simulink model "Vehicle_Model_Controller_Feb25"  (R2020b)
settings: Solver=VariableStepAuto  StartTime=0.0  StopTime=60  FixedStep=0.015  MaxStep=0.015  RelTol=1e-3
model workspace (MAT data in the model file):
  Kp = 10
  understeer_gradient = 0.05
values from neighbouring files (symbols this model uses):
  I = 0    [startup.m]
  P = 10    [startup.m]
  T = 0    [startup.m]
undefined symbols (not defined in the file or in its folder): DiscIntNeverNeededParam
libraries: fl_lib x32, nesl_utility x24, sdl_lib x8, vehdynlibsteering x1, autolibshared x1, autolibdatasheetbattery x1, pid_lib x1
(part 1 of 3)
settings Model: TunableVars=F_sv,F_x_ij,F_x_ij_max,F_y_fl,F_y_fr,F_y_ij,F_y_rl,F_y_rr,J_z,K_1,K_2,LB,PID,R,T_x_ij,UP,delta,driver_input,err,l,l_f,l_r,linsol,s,s_f,s_r,x,x_1,x_2,x_3,x_4,y,y_1,y_2,y_3,y_4  TunableVarsStorageClass=Auto,Auto,Auto,Auto,Auto,Auto,Auto,Auto,Auto,Auto,Auto,Auto,Auto,Auto,Auto,Auto,Auto,Auto,Auto,Auto,Auto,Auto,Auto,Auto,Auto,Auto,Auto,Auto,Auto,Auto,Auto,Auto,Auto,Auto,Auto,Auto  TunableVarsTypeQualifier=,,,,,,,,,,,,,,,,,,,,,,,,,,,,,,,,,,,  ParameterArgumentNames=understeer_gradient  OrderedModelArguments=off  Creator=True  LastModifiedBy=Inver
settings SolverCC: MaxConsecutiveMinStep=10  AutoInsertRateTranBlk=on  MinimalZcImpactIntegration=on
settings DataIOCC: ExternalInput=Sheet1.getElement('driver_input'),Sheet1.getElement('P_A'),Sheet1.getElement('B_A'),Sheet1.getElement('steering_angle'),Sheet1.getElement('wind x'),Sheet1.getElement('wind y'),Sheet1.getElement('wind z'),Sheet1.getElement('batt_temp')  LoadExternalInput=on
settings OptimizationCC: DefaultParameterBehavior=Inlined  UseFloatMulNetSlope=on  InlineInvariantSignals=on  BufferReuse=off  EnhancedBackFolding=on  PassReuseOutputArgsThreshold=0  EfficientFloat2IntCast=on  EfficientMapNaN2IntZero=off  OptimizeBlockOrder=speed  DifferentSizesBufferReuse=on
settings DebuggingCC: RTPrefix=warning  ReadBeforeWriteMsg=DisableAll  WriteAfterWriteMsg=DisableAll  WriteAfterReadMsg=DisableAll  SolverPrmCheckMsg=error  MultiTaskDSMMsg=none  ParameterTunabilityLossMsg=error  ArithmeticOperatorsInVariantConditions=warning
settings HardwareCC: TargetBitPerPointer=64  TargetBitPerSizeT=64  TargetBitPerPtrDiffT=64  TargetLongLongMode=on  TargetIntDivRoundTo=Zero  TargetEndianess=LittleEndian  TargetWordSize=64  TargetHWDeviceType=MATLAB Host  ProdEqTarget=off
settings ModelReferenceCC: UpdateModelReferenceTargets=IfOutOfDate
settings SFSimCC: SimCustomHeaderCode="#include \"bigM_v2_func.h\""  SimUserSources=bigM_v2_func.c  SimUserIncludeDirs=$matlabroot$\toolbox\rtw\rtwdemos\EmbeddedCoderOverview\  SFSimEcho=off  CustomCodeUndefinedFunction=UseInterfaceOnly
settings RTWCC: Description=Rapid Simulation Target  SystemTargetFile=rsim.tlc  GenCodeOnly=on  TemplateMakefile=rsim_default_tmf  GenerateReport=on  BuildConfiguration=Faster Runs  LaunchReport=on  CheckMdlBeforeBuild=Warning
settings CodeAppCC: ForceParamTrailComments=on  OperatorAnnotations=on
settings RSimTargetCC: TargetLangStandard=C99 (ISO)
settings ConfigComp: CovScope=ReferencedModels  DVMaxProcessTime=100  DVTestSuiteOptimization=CombinedObjectives (Nonlinear Extended)  DVDetectOutOfBounds=on
settings SimscapeCC: SimscapeLogType=local

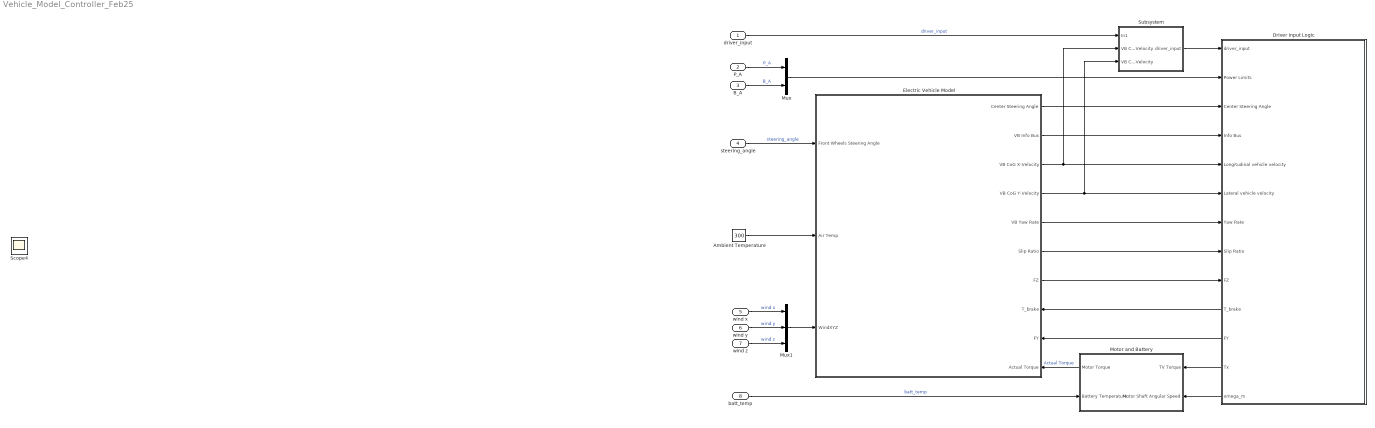
== system Vehicle_Model_Controller_Feb25 ==
  driver_input : Inport  Interpolate=off
  P_A : Inport  Port=2  Interpolate=off
  B_A : Inport  Port=3  Interpolate=off
  steering_angle : Inport  Port=4  Interpolate=off
  wind x : Inport  Port=5  Interpolate=off
  wind y : Inport  Port=6  Interpolate=off
  wind z : Inport  Port=7  Interpolate=off
  batt_temp : Inport  Port=8  Interpolate=off
  Ambient Temperature : Constant  Value=300
  Driver Input Logic : Subsystem
      settings: PortSchema="{\"entries\":[{\"content\":{\"sides\":[{\"content\":{\"connectorIds\":[\"In1\",\"In2\",\"In3\",\"In4\",\"In5\",\"In6\",\"In7\",\"In8\",\"In9\",\"Out1\",\"Out2\",\"Out3\",\"Out4\"]},\"type\":\"ConnectorPlacement.EquallySpacedRectSide\",\"uuid\":\"60aa76ce-4868-40a7-a4fe-105a8e1f1745\"},{\"content\":{\"connectorIds\":[],\"side\":\"RIGHT\"},\"type\":\"ConnectorPlacement.EquallySpacedRectSide\",\"uuid\":\"32a33737-884d-4b24-9f96-3d3edd17fbca\"},{\"content\":{\"connectorIds\":[],\"side\":\"TOP\"},\"type\":\"ConnectorPlacement.EquallySpacedRectSide\",\"uuid\":\"827704d2-5b88-4535-b448-6dd72aa29b4b\"},{\"content\":{\"connectorIds\":[],\"side\":\"BOTTOM\"},\"type\":\"ConnectorPlacement.EquallySpacedRectSide\",\"uuid\":\"278cc67c-48ea-4083-b722-927ef88660f9\"},{\"content\":{\"connectorIds\":[],\"side\":\"HIDDEN\"},\"type\":\"ConnectorPlacement.EquallySpacedRectSide\",\"uuid\":\"0c403b58-0099-4716-b0b3-86e3ff44a502\"}]},\"type\":\"ConnectorPlacement.EquallySpacedConnector\",\"uuid\":\"f0e3ee49-9104-4d68-bbfb-d96c82f46588\"}],\"packageUris\":[\"http://schema.mathworks.com/mf0/Connector/R2020b\"],\"version\":\"1.0\"}"
  Electric Vehicle Model : Subsystem
      settings: PortSchema="{\"entries\":[{\"content\":{\"sides\":[{\"content\":{\"connectorIds\":[\"In1\",\"In2\",\"In3\"]},\"type\":\"ConnectorPlacement.EquallySpacedRectSide\",\"uuid\":\"d948e6fd-2a7c-48d4-af15-7a99a175752d\"},{\"content\":{\"connectorIds\":[\"Out1\",\"Out2\",\"Out3\",\"Out4\",\"Out5\",\"Out6\",\"Out7\",\"In4\",\"In5\",\"In6\"],\"side\":\"RIGHT\"},\"type\":\"ConnectorPlacement.EquallySpacedRectSide\",\"uuid\":\"1a47e5e8-2455-404d-921d-9ae775b78aa8\"},{\"content\":{\"connectorIds\":[],\"side\":\"TOP\"},\"type\":\"ConnectorPlacement.EquallySpacedRectSide\",\"uuid\":\"f91bd10b-9e07-4da1-95e5-01fed64ff2a2\"},{\"content\":{\"connectorIds\":[],\"side\":\"BOTTOM\"},\"type\":\"ConnectorPlacement.EquallySpacedRectSide\",\"uuid\":\"a21defd9-60a5-4926-b7a0-aedbd24b2311\"},{\"content\":{\"connectorIds\":[],\"side\":\"HIDDEN\"},\"type\":\"ConnectorPlacement.EquallySpacedRectSide\",\"uuid\":\"26c45b26-0233-46e7-86a3-2b3d6a7840e5\"}]},\"type\":\"ConnectorPlacement.EquallySpacedConnector\",\"uuid\":\"a0d97086-54ab-4f92-bc82-b1adaed3f48d\"}],\"packageUris\":[\"http://schema.mathworks.com/mf0/Connector/R2020b\"],\"version\":\"1.0\"}"
  Motor and Battery : Subsystem
      settings: PortSchema="{\"entries\":[{\"content\":{\"sides\":[{\"content\":{\"connectorIds\":[\"Out1\",\"In1\"]},\"type\":\"ConnectorPlacement.EquallySpacedRectSide\",\"uuid\":\"0a1f914b-70eb-46fa-9e3d-552685e5145b\"},{\"content\":{\"connectorIds\":[\"In2\",\"In3\"],\"side\":\"RIGHT\"},\"type\":\"ConnectorPlacement.EquallySpacedRectSide\",\"uuid\":\"3f4913ad-53b1-4c2d-9942-63851d66d84d\"},{\"content\":{\"connectorIds\":[],\"side\":\"TOP\"},\"type\":\"ConnectorPlacement.EquallySpacedRectSide\",\"uuid\":\"355326fa-9c02-45e7-a319-d2a0d6b3d4bd\"},{\"content\":{\"connectorIds\":[],\"side\":\"HIDDEN\"},\"type\":\"ConnectorPlacement.EquallySpacedRectSide\",\"uuid\":\"65af7ff0-f0aa-4be0-a188-dc3dcb8956e6\"}]},\"type\":\"ConnectorPlacement.EquallySpacedConnector\",\"uuid\":\"023a46d9-a637-4c8e-84c1-6893dcef87c2\"}],\"packageUris\":[\"http://schema.mathworks.com/mf0/Connector/R2020b\"],\"version\":\"1.0\"}"
  Mux : Mux  Inputs=2
  Mux1 : Mux  Inputs=3
  Subsystem : Subsystem
  Scope4 : Scope
  wires:
  Ambient Temperature/1 -> Electric Vehicle Model/2(Air Temp)
  Electric Vehicle Model/2(VB Info Bus) -> Driver Input Logic/4(Info Bus)
  Electric Vehicle Model/3(VB CoG X-Velocity) -> Subsystem/2(VB CoG X-Velocity), Driver Input Logic/5(Longitudinal vehicle velocity)
  Electric Vehicle Model/4(VB CoG Y-Velocity) -> Subsystem/3(VB CoG Y-Velocity), Driver Input Logic/6(Lateral vehicle velocity)
  Electric Vehicle Model/5(VB Yaw Rate) -> Driver Input Logic/7(Yaw Rate)
  wind x/1 -> Mux1/1  "wind x"
  wind y/1 -> Mux1/2  "wind y"
  wind z/1 -> Mux1/3  "wind z"
  Mux1/1 -> Electric Vehicle Model/3(WindXYZ)
  batt_temp/1 -> Motor and Battery/1(Battery Temperature)  "batt_temp"
  steering_angle/1 -> Electric Vehicle Model/1(Front Wheels Steering Angle)  "steering_angle"
  Electric Vehicle Model/1(Center Steering Angle) -> Driver Input Logic/3(Center Steering Angle)
  Driver Input Logic/4(omega_m) -> Motor and Battery/3(Motor Shaft Angular Speed)
  Driver Input Logic/3(Tx) -> Motor and Battery/2(TV Torque)
  Mux/1 -> Driver Input Logic/2(Power Limits)
  P_A/1 -> Mux/1  "P_A"
  B_A/1 -> Mux/2  "B_A"
  Driver Input Logic/1(T_brake) -> Electric Vehicle Model/4(T_brake)
  Electric Vehicle Model/6(Slip Ratio) -> Driver Input Logic/8(Slip Ratio)
  Electric Vehicle Model/7(FZ) -> Driver Input Logic/9(FZ)
  Driver Input Logic/2(FY) -> Electric Vehicle Model/5(FY)
  Motor and Battery/1(Motor Torque) -> Electric Vehicle Model/6(Actual Torque)  "Actual Torque"
  Subsystem/1(driver_input) -> Driver Input Logic/1(driver_input)
  driver_input/1 -> Subsystem/1(In1)  "driver_input"

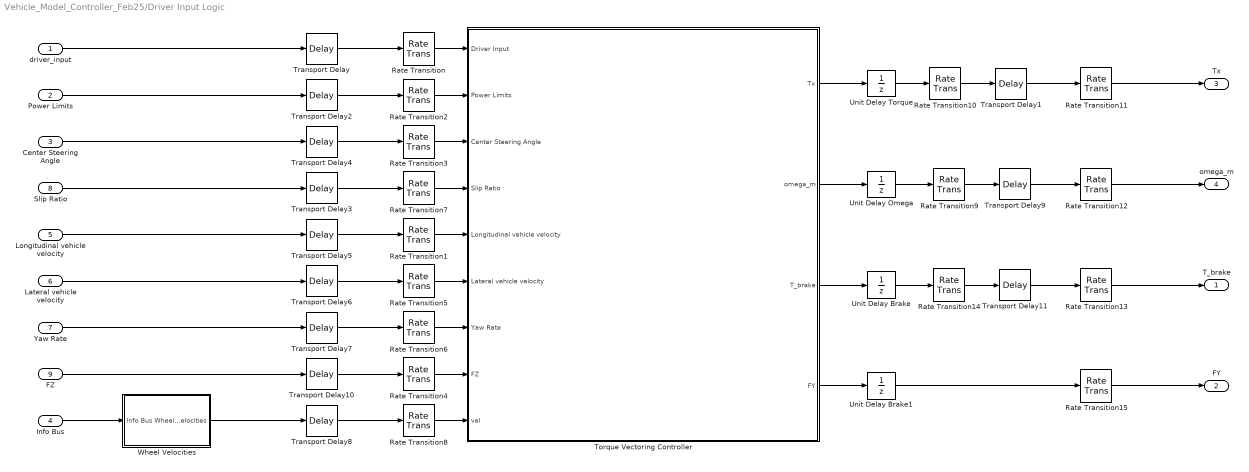
== system Vehicle_Model_Controller_Feb25/Driver Input Logic ==
  driver_input : Inport
  Power Limits : Inport  Port=2
  Center Steering Angle : Inport  Port=3
  Info Bus : Inport  Port=4
  Longitudinal vehicle velocity : Inport  Port=5
  Lateral vehicle velocity : Inport  Port=6
  Yaw Rate : Inport  Port=7
  Slip Ratio : Inport  Port=8
  FZ : Inport  Port=9
  " Wheel Velocities" : Subsystem
  Rate Transition{,1,3,5..6,11} (6 alike) : RateTransition  OutPortSampleTime=0.015
  Rate Transition10 : RateTransition  OutPortSampleTime=0
  Rate Transition{7,12..13,15} (4 alike) : RateTransition  InitialCondition=[0 0 0 0]  OutPortSampleTime=0.015
  Rate Transition14 : RateTransition  InitialCondition=[0 0 0 0]  OutPortSampleTime=0
  Rate Transition2 : RateTransition  InitialCondition=[0 0]  OutPortSampleTime=0.015
  Rate Transition4 : RateTransition  InitialCondition=[450 450 450 450]  OutPortSampleTime=0.015
  Rate Transition8 : RateTransition  InitialCondition=[0 0 0 0 0 0]  OutPortSampleTime=0.015
  Rate Transition9 : RateTransition  InitialCondition=[0 0 0 0]  OutPortSampleTime=0
  Torque Vectoring Controller : Subsystem
  Transport Delay{,4..7} (5 alike) : TransportDelay  DelayTime=0.015  BufferSize=25000
  Transport Delay1 : TransportDelay  DelayTime=0.007  InitialOutput=[0; 0; 0; 0]  BufferSize=25000
  Transport Delay10 : TransportDelay  DelayTime=0.015  InitialOutput=[0 0 0 0]  BufferSize=25000
  Transport Delay11 : TransportDelay  DelayTime=0.007  InitialOutput=[0 0 0 0]  BufferSize=25000
  Transport Delay2 : TransportDelay  DelayTime=0.015  InitialOutput=[0 0]  BufferSize=25000
  Transport Delay3 : TransportDelay  DelayTime=0.015  InitialOutput=[0 0 0 0]  BufferSize=25000
  Transport Delay8 : TransportDelay  DelayTime=0.015  InitialOutput=[0 0 0 0 0 0]  BufferSize=25000
  Transport Delay9 : TransportDelay  DelayTime=0.007  InitialOutput=[0 0 0 0]  BufferSize=25000
  Unit Delay Brake : UnitDelay  InitialCondition=[0, 0, 0, 0]  SampleTime=-1  HasFrameUpgradeWarning=on
  Unit Delay Brake1 : UnitDelay  InitialCondition=[0, 0, 0, 0]  SampleTime=-1  HasFrameUpgradeWarning=on
  Unit Delay Omega : UnitDelay  InitialCondition=[0, 0, 0, 0]  SampleTime=-1  HasFrameUpgradeWarning=on
  Unit Delay Torque : UnitDelay  InitialCondition=[0; 0; 0; 0]  SampleTime=-1  HasFrameUpgradeWarning=on
  T_brake : Outport
  FY : Outport  Port=2
  Tx : Outport  Port=3
  omega_m : Outport  Port=4
  wires:
  Rate Transition/1 -> Torque Vectoring Controller/1(Driver Input)
  Rate Transition2/1 -> Torque Vectoring Controller/2(Power Limits)
  Rate Transition6/1 -> Torque Vectoring Controller/7(Yaw Rate)
  Rate Transition5/1 -> Torque Vectoring Controller/6(Lateral vehicle velocity)
  Rate Transition1/1 -> Torque Vectoring Controller/5(Longitudinal vehicle velocity)
  Rate Transition3/1 -> Torque Vectoring Controller/3(Center Steering Angle)
  Rate Transition7/1 -> Torque Vectoring Controller/4(Slip Ratio)
  Info Bus/1 -> " Wheel Velocities"/1(Info Bus)
  Rate Transition4/1 -> Torque Vectoring Controller/8(FZ)
  Rate Transition8/1 -> Torque Vectoring Controller/9(vel)
  Rate Transition9/1 -> Transport Delay9/1
  Unit Delay Omega/1 -> Rate Transition9/1
  Torque Vectoring Controller/1(Tx) -> Unit Delay Torque/1
  Rate Transition12/1 -> omega_m/1
  Torque Vectoring Controller/2(omega_m) -> Unit Delay Omega/1
  Torque Vectoring Controller/3(T_brake) -> Unit Delay Brake/1
  Transport Delay/1 -> Rate Transition/1
  driver_input/1 -> Transport Delay/1
  Transport Delay6/1 -> Rate Transition5/1
  Transport Delay5/1 -> Rate Transition1/1
  Transport Delay3/1 -> Rate Transition7/1
  Transport Delay4/1 -> Rate Transition3/1
  Transport Delay2/1 -> Rate Transition2/1
  Power Limits/1 -> Transport Delay2/1
  Center Steering Angle/1 -> Transport Delay4/1
  Slip Ratio/1 -> Transport Delay3/1
  Longitudinal vehicle velocity/1 -> Transport Delay5/1
  Lateral vehicle velocity/1 -> Transport Delay6/1
  Transport Delay7/1 -> Rate Transition6/1
  Yaw Rate/1 -> Transport Delay7/1
  Transport Delay8/1 -> Rate Transition8/1
  " Wheel Velocities"/1(Wheel Velocities) -> Transport Delay8/1
  Unit Delay Torque/1 -> Rate Transition10/1
  Rate Transition10/1 -> Transport Delay1/1
  Transport Delay1/1 -> Rate Transition11/1
  Rate Transition11/1 -> Tx/1
  Transport Delay9/1 -> Rate Transition12/1
  Transport Delay11/1 -> Rate Transition13/1
  Rate Transition14/1 -> Transport Delay11/1
  Rate Transition13/1 -> T_brake/1
  Unit Delay Brake/1 -> Rate Transition14/1
  Transport Delay10/1 -> Rate Transition4/1
  FZ/1 -> Transport Delay10/1
  Unit Delay Brake1/1 -> Rate Transition15/1
  Torque Vectoring Controller/4(FY) -> Unit Delay Brake1/1
  Rate Transition15/1 -> FY/1

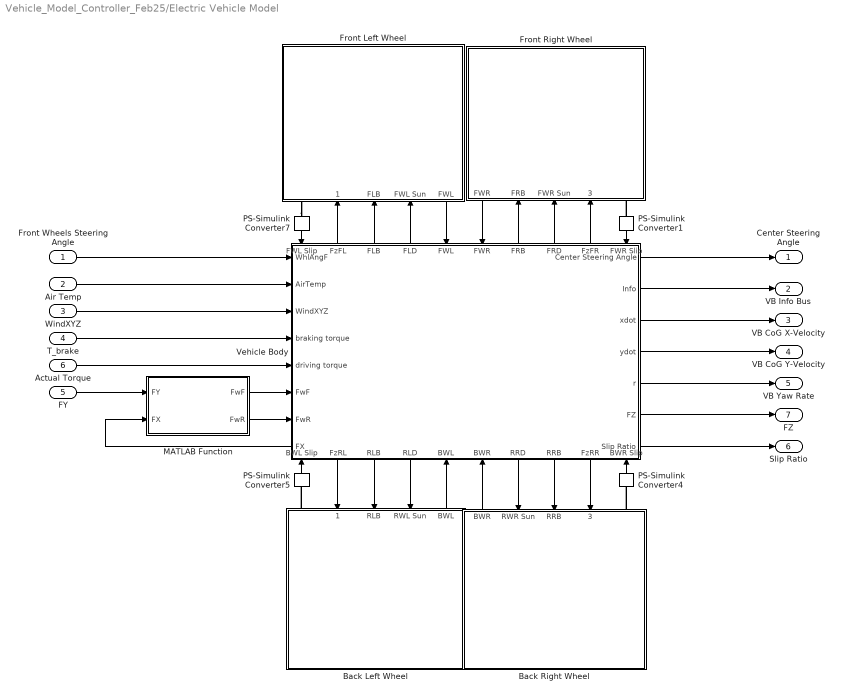
== system Vehicle_Model_Controller_Feb25/Electric Vehicle Model ==
  Front Wheels Steering Angle : Inport
  Air Temp : Inport  Port=2
  WindXYZ : Inport  Port=3
  T_brake : Inport  Port=4
  FY : Inport  Port=5
  Actual Torque : Inport  Port=6
  Back Left Wheel : Subsystem
      settings: PortSchema="{\"entries\":[{\"content\":{\"sides\":[{\"content\":{\"connectorIds\":[]},\"type\":\"ConnectorPlacement.EquallySpacedRectSide\",\"uuid\":\"2b71f4a5-a413-4669-bce9-c022c008b37f\"},{\"content\":{\"connectorIds\":[],\"side\":\"RIGHT\"},\"type\":\"ConnectorPlacement.EquallySpacedRectSide\",\"uuid\":\"bc97bf18-1824-4dcb-a7bf-b21d223b914e\"},{\"content\":{\"connectorIds\":[\"LConn1\",\"In1\",\"In2\",\"In3\",\"Out1\"],\"side\":\"TOP\"},\"type\":\"ConnectorPlacement.EquallySpacedRectSide\",\"uuid\":\"45ab5d46-9661-4401-8349-74a293812c9f\"},{\"content\":{\"connectorIds\":[],\"side\":\"HIDDEN\"},\"type\":\"ConnectorPlacement.EquallySpacedRectSide\",\"uuid\":\"98f7b348-3a36-4ee3-a398-c35d25fd5096\"}]},\"type\":\"ConnectorPlacement.EquallySpacedConnector\",\"uuid\":\"08ca7540-1c7d-4720-99bc-9cfb6f12d06d\"}],\"packageUris\":[\"http://schema.mathworks.com/mf0/Connector/R2020b\"],\"version\":\"1.0\"}"
  Back Right Wheel : Subsystem
      settings: PortSchema="{\"entries\":[{\"content\":{\"sides\":[{\"content\":{\"connectorIds\":[]},\"type\":\"ConnectorPlacement.EquallySpacedRectSide\",\"uuid\":\"0dce7c84-f49c-47da-a985-42537e31f80d\"},{\"content\":{\"connectorIds\":[],\"side\":\"RIGHT\"},\"type\":\"ConnectorPlacement.EquallySpacedRectSide\",\"uuid\":\"6a2d686c-11f7-455f-a903-3ea36dc1e6c4\"},{\"content\":{\"connectorIds\":[\"Out1\",\"In1\",\"In2\",\"In3\",\"LConn1\"],\"side\":\"TOP\"},\"type\":\"ConnectorPlacement.EquallySpacedRectSide\",\"uuid\":\"f7c89490-d7ec-4842-8f49-6b07ecd893d9\"},{\"content\":{\"connectorIds\":[],\"side\":\"HIDDEN\"},\"type\":\"ConnectorPlacement.EquallySpacedRectSide\",\"uuid\":\"1095a815-35e8-40c4-8518-dd6454b2f370\"}]},\"type\":\"ConnectorPlacement.EquallySpacedConnector\",\"uuid\":\"2c7105c5-1f43-4c21-98a2-86270cd61bf9\"}],\"packageUris\":[\"http://schema.mathworks.com/mf0/Connector/R2020b\"],\"version\":\"1.0\"}"
  Front Left Wheel : Subsystem
      settings: PortSchema="{\"entries\":[{\"content\":{\"sides\":[{\"content\":{\"connectorIds\":[]},\"type\":\"ConnectorPlacement.EquallySpacedRectSide\",\"uuid\":\"2b71f4a5-a413-4669-bce9-c022c008b37f\"},{\"content\":{\"connectorIds\":[],\"side\":\"RIGHT\"},\"type\":\"ConnectorPlacement.EquallySpacedRectSide\",\"uuid\":\"bc97bf18-1824-4dcb-a7bf-b21d223b914e\"},{\"content\":{\"connectorIds\":[],\"side\":\"TOP\"},\"type\":\"ConnectorPlacement.EquallySpacedRectSide\",\"uuid\":\"45ab5d46-9661-4401-8349-74a293812c9f\"},{\"content\":{\"connectorIds\":[\"RConn1\",\"In1\",\"In2\",\"In3\",\"Out1\"],\"side\":\"BOTTOM\"},\"type\":\"ConnectorPlacement.EquallySpacedRectSide\",\"uuid\":\"626a829b-c6a7-44fa-8f29-1d2c0438f6d4\"},{\"content\":{\"connectorIds\":[],\"side\":\"HIDDEN\"},\"type\":\"ConnectorPlacement.EquallySpacedRectSide\",\"uuid\":\"98f7b348-3a36-4ee3-a398-c35d25fd5096\"}]},\"type\":\"ConnectorPlacement.EquallySpacedConnector\",\"uuid\":\"08ca7540-1c7d-4720-99bc-9cfb6f12d06d\"}],\"packageUris\":[\"http://schema.mathworks.com/mf0/Connector/R2020b\"],\"version\":\"1.0\"}"
  Front Right Wheel : Subsystem
      settings: PortSchema="{\"entries\":[{\"content\":{\"sides\":[{\"content\":{\"connectorIds\":[]},\"type\":\"ConnectorPlacement.EquallySpacedRectSide\",\"uuid\":\"0dce7c84-f49c-47da-a985-42537e31f80d\"},{\"content\":{\"connectorIds\":[],\"side\":\"RIGHT\"},\"type\":\"ConnectorPlacement.EquallySpacedRectSide\",\"uuid\":\"6a2d686c-11f7-455f-a903-3ea36dc1e6c4\"},{\"content\":{\"connectorIds\":[],\"side\":\"TOP\"},\"type\":\"ConnectorPlacement.EquallySpacedRectSide\",\"uuid\":\"f7c89490-d7ec-4842-8f49-6b07ecd893d9\"},{\"content\":{\"connectorIds\":[\"Out1\",\"In1\",\"In2\",\"In3\",\"RConn1\"],\"side\":\"BOTTOM\"},\"type\":\"ConnectorPlacement.EquallySpacedRectSide\",\"uuid\":\"41036381-c0f5-4b34-b4f9-9bf6c3122150\"},{\"content\":{\"connectorIds\":[],\"side\":\"HIDDEN\"},\"type\":\"ConnectorPlacement.EquallySpacedRectSide\",\"uuid\":\"1095a815-35e8-40c4-8518-dd6454b2f370\"}]},\"type\":\"ConnectorPlacement.EquallySpacedConnector\",\"uuid\":\"2c7105c5-1f43-4c21-98a2-86270cd61bf9\"}],\"packageUris\":[\"http://schema.mathworks.com/mf0/Connector/R2020b\"],\"version\":\"1.0\"}"
  MATLAB Function : MATLAB Function  TreatAsAtomicUnit=on
  PS-Simulink Converter{1,4..5,7} (4 alike) : nesl_utility/PS-Simulink Converter  PhysicalDomain=network_engine_domain  SubClassName=ps_output  LeftPortType=input  RightPortType=output  PseudoPeriodic=off  Frequencies=[]  Unit=inherit  AffineConversion=off
      settings: SourceProductBaseCode=PW,SS
  Vehicle Body : Subsystem
      settings: PortSchema="{\"entries\":[{\"content\":{\"sides\":[{\"content\":{\"connectorIds\":[\"In1\",\"In2\",\"In3\",\"In4\",\"In5\",\"In6\",\"In7\",\"Out20\"]},\"type\":\"ConnectorPlacement.EquallySpacedRectSide\",\"uuid\":\"603222f6-0091-4ad0-bf19-39b4be84e01e\"},{\"content\":{\"connectorIds\":[\"Out1\",\"Out2\",\"Out3\",\"Out4\",\"Out5\",\"Out6\",\"Out7\"],\"side\":\"RIGHT\"},\"type\":\"ConnectorPlacement.EquallySpacedRectSide\",\"uuid\":\"c4db7259-b5a3-4868-8718-dda29d48254f\"},{\"content\":{\"connectorIds\":[\"In8\",\"Out14\",\"Out15\",\"Out16\",\"In9\",\"In10\",\"Out17\",\"Out18\",\"Out19\",\"In11\"],\"side\":\"TOP\"},\"type\":\"ConnectorPlacement.EquallySpacedRectSide\",\"uuid\":\"a713a325-471a-4f93-96c3-fb024f273799\"},{\"content\":{\"connectorIds\":[\"In12\",\"Out8\",\"Out9\",\"Out10\",\"In13\",\"In14\",\"Out11\",\"Out12\",\"Out13\",\"In15\"],\"side\":\"BOTTOM\"},\"type\":\"ConnectorPlacement.EquallySpacedRectSide\",\"uuid\":\"12db6ab3-ce51-4037-9ece-8ccfa03e22af\"},{\"content\":{\"connectorIds\":[],\"side\":\"HIDDEN\"},\"type\":\"ConnectorPlacement.EquallySpacedRectSide\",\"uuid\":\"dd051903-611f-41d3-87ac-1430d6d99127\"}]},\"type\":\"ConnectorPlacement.EquallySpacedConnector\",\"uuid\":\"5fd2346c-a877-48e3-8a05-bb1d13d3d04b\"}],\"packageUris\":[\"http://schema.mathworks.com/mf0/Connector/R2020b\"],\"version\":\"1.0\"}"
  Center Steering Angle : Outport
  VB Info Bus : Outport  Port=2
  VB CoG X-Velocity : Outport  Port=3
  VB CoG Y-Velocity : Outport  Port=4
  VB Yaw Rate : Outport  Port=5
  Slip Ratio : Outport  Port=6
  FZ : Outport  Port=7
  wires:
  Vehicle Body/14(FzFL) -> Front Left Wheel/1(FWL Normal)
  PS-Simulink Converter5/1 -> Vehicle Body/12(BWL Slip)
  Vehicle Body/5(r) -> VB Yaw Rate/1
  PS-Simulink Converter4/1 -> Vehicle Body/15(BWR Slip)
  Vehicle Body/8(FzRL) -> Back Left Wheel/1(RWL Normal)
  Vehicle Body/13(FzRR) -> Back Right Wheel/3(BWR Normal)
  Air Temp/1 -> Vehicle Body/2(AirTemp)
  WindXYZ/1 -> Vehicle Body/3(WindXYZ)
  Vehicle Body/3(xdot) -> VB CoG X-Velocity/1
  Vehicle Body/2(Info) -> VB Info Bus/1
  Vehicle Body/19(FzFR) -> Front Right Wheel/3(FWR Normal)
  Vehicle Body/4(ydot) -> VB CoG Y-Velocity/1
  Vehicle Body/1(Center Steering Angle) -> Center Steering Angle/1
  Front Wheels Steering Angle/1 -> Vehicle Body/1(WhlAngF)
  Vehicle Body/16(FLD) -> Front Left Wheel/3(FWL Sun)
  Vehicle Body/18(FRD) -> Front Right Wheel/2(FWR Sun)
  Vehicle Body/15(FLB) -> Front Left Wheel/2(FLB)
  Vehicle Body/17(FRB) -> Front Right Wheel/1(FRB)
  PS-Simulink Converter7/1 -> Vehicle Body/8(FWL Slip)
  Vehicle Body/7(Slip Ratio) -> Slip Ratio/1
  PS-Simulink Converter1/1 -> Vehicle Body/11(FWR Slip)
  Vehicle Body/6(FZ) -> FZ/1
  MATLAB Function/2(FwR) -> Vehicle Body/7(FwR)
  FY/1 -> MATLAB Function/1(FY)
  MATLAB Function/1(FwF) -> Vehicle Body/6(FwF)
  Vehicle Body/9(RLB) -> Back Left Wheel/2(RLB)
  Vehicle Body/12(RRB) -> Back Right Wheel/2(RRB)
  Vehicle Body/10(RLD) -> Back Left Wheel/3(RWL Sun)
  Vehicle Body/11(RRD) -> Back Right Wheel/1(RWR Sun)
  Back Right Wheel/1(BWR) -> Vehicle Body/14(BWR)
  Back Left Wheel/1(BWL) -> Vehicle Body/13(BWL)
  Front Left Wheel/1(FWL) -> Vehicle Body/9(FWL)
  Front Right Wheel/1(FWR) -> Vehicle Body/10(FWR)
  T_brake/1 -> Vehicle Body/4(braking torque)
  Actual Torque/1 -> Vehicle Body/5(driving torque)
  Vehicle Body/20(FX) -> MATLAB Function/2(FX)
  connections:
  Front Left Wheel/RConn1 -- PS-Simulink Converter7/LConn1
  Back Right Wheel/LConn1 -- PS-Simulink Converter4/LConn1
  Back Left Wheel/LConn1 -- PS-Simulink Converter5/LConn1
  PS-Simulink Converter1/LConn1 -- Front Right Wheel/RConn1

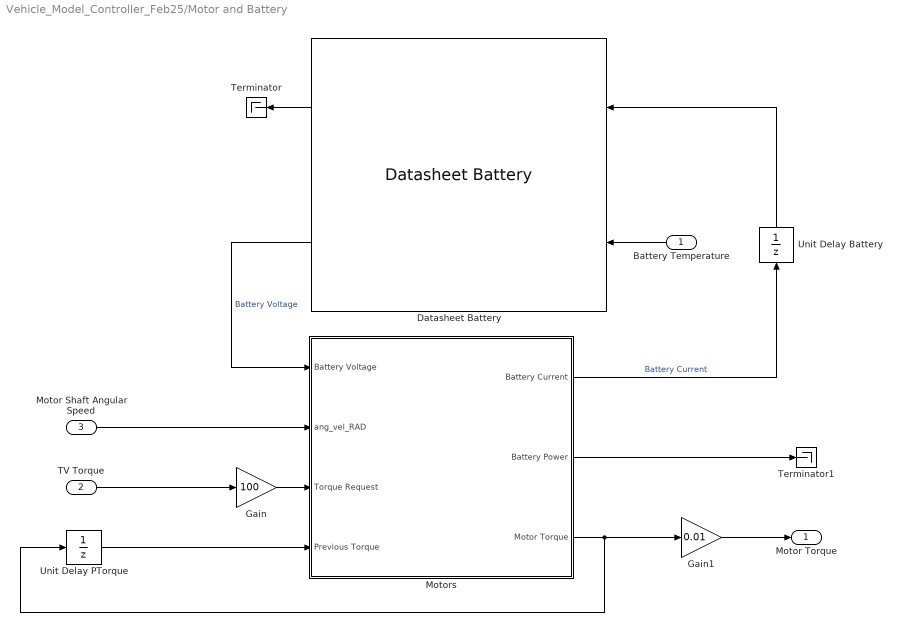
== system Vehicle_Model_Controller_Feb25/Motor and Battery ==
  Battery Temperature : Inport
  TV Torque : Inport  Port=2
  Motor Shaft Angular Speed : Inport  Port=3
  Datasheet Battery : autolibdatasheetbattery/Datasheet Battery  CapacityCtrl=Parameter  OutputVlt=Unfiltered  BattChargeMax=32.5  Em=[2.8 3.228 3.284 3.361 3.408 3.427 3.472 3.477 3.493 3.504 3.516 3.528 3.537 3.545 3.555 3.561 3.566 3.576 3.587 3.589 3.594 3.6 3.608 3.61 3.616 3.619 3.626 3.632 3.637 3.64 3.645 3.646 3.652 3.655 3.658 3.661 3.664 3.668 3.673 3.678 3.68 3.681 3.686 3.692 3.699 3.702 3.705 3.71 3.717 3.723 3.728 3.733 3.735 3.742 3.749 3.755 3.761 3.768 3.773 3.78 3.791 3.798 3.798 3.814 3.818 3.825 3.841 3.846 3.855 3.863 3.877 3.885 3.894 3.907 3.919 3.926 3.935 3.944 3.954 3.964 3.974 3.988 3.998 4.014 4.029 4.034 4.047 4.065 4.074 4.086 4.097 4.131 4.126 4.138 4.15 4.18 4.174 4.187 4.207 4.231 4.221]  CapLUTBp=[0 0.01 0.02 0.03 0.04 0.05 0.06 0.07 0.08 0.09 0.1 0.11 0.12 0.13 0.14 0.15 0.16 0.17 0.18 0.19 0.2 0.21 0.22 0.23 0.24 0.25 0.26 0.27 0.28 0.29 0.3 0.31 0.32 0.33 0.34 0.35 0.36 0.37 0.38 0.39 0.4 0.41 0.42 0.43 0.44 0.45 0.46 0.47 0.48 0.49 0.5 0.51 0.52 0.53 0.54 0.55 0.56 0.57 0.58 0.59 0.6 0.61 0.62 0.63 0.64 0.65 0.66 0.67 0.68 0.69 0.7 0.71 0.72 0.73 0.74 0.75 0.76 0.77 0.78 0.79 0.8 0.81 0.82 0.83 0.84 0.85 0.86 0.87 0.88 0.89 0.9 0.91 0.92 0.93 0.94 0.95 0.96 0.97 0.98 0.99 1]  RInt=[0.008846 0.009319 0.009027 0.00847 0.01032 0.01314;0.006389 0.006554 0.005553 0.005525 0.006043 0.007805;0.004364 0.004101 0.00406 0.003452 0.003846 0.004517;0.002031 0.002563 0.002532 0.00246 0.002716 0.003047;0.001443 0.001825 0.001795 0.001778 0.001924 0.002234;0.0005603 0.0007192 0.0006887 0.0007557 0.0007355 0.001014;0.001028 0.001338 0.001 0.001536 0.001546 0.002789]  BattTempBp=[243.1 253.1 263.1 273.1 283.1 298.1 313.1]  CapSOCBp=[0 0.2 0.4 0.6 0.8 1]  Ns=81  Np=2  BattCapInit=26  Tc=1/1000  Vinit=4.221  RefBlkName='autolibdatasheetbattery/Datasheet Battery'
      settings: SourceProductBaseCode=PW
  Gain : Gain  Gain=100
  Gain1 : Gain  Gain=0.01
  Motors : Subsystem
  Terminator : Terminator
  Terminator1 : Terminator
  Unit Delay Battery : UnitDelay  SampleTime=-1  HasFrameUpgradeWarning=on
  Unit Delay PTorque : UnitDelay  InitialCondition=[0, 0, 0, 0]  SampleTime=-1  HasFrameUpgradeWarning=on
  Motor Torque : Outport
  wires:
  Datasheet Battery/1 -> Terminator/1
  Battery Temperature/1 -> Datasheet Battery/2
  Unit Delay Battery/1 -> Datasheet Battery/1
  Motors/1(Battery Current) -> Unit Delay Battery/1  "Battery Current"
  Gain/1 -> Motors/3(Torque Request)
  Gain1/1 -> Motor Torque/1
  Motors/3(Motor Torque) -> Unit Delay PTorque/1, Gain1/1
  Motors/2(Battery Power) -> Terminator1/1
  Datasheet Battery/2 -> Motors/1(Battery Voltage)  "Battery Voltage"
  Unit Delay PTorque/1 -> Motors/4(Previous Torque)
  TV Torque/1 -> Gain/1
  Motor Shaft Angular Speed/1 -> Motors/2(ang_vel_RAD)

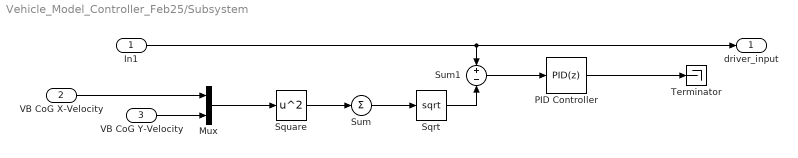
== system Vehicle_Model_Controller_Feb25/Subsystem ==
  In1 : Inport
  VB CoG X-Velocity : Inport  Port=2
  VB CoG Y-Velocity : Inport  Port=3
  Mux : Mux  Inputs=2
  PID Controller : pid_lib/PID Controller  Controller=PID  Form=Parallel  TimeDomain=Discrete-time  UseExternalTs=off  SampleTime=-1  IntegratorMethod=Forward Euler  FilterMethod=Forward Euler  ControllerParametersSource=internal  P=0.4  I=0.5  D=0  UseFilter=on  N=100  TunerSelectOption=Transfer Function Based (PID Tuner App)  InitialConditionSource=internal  InitialConditionForIntegrator=0  InitialConditionForFilter=0  DifferentiatorICPrevScaledInput=0  ExternalReset=none  TrackingMode=off  Kt=1  LimitOutput=on  SatLimitsSource=internal  UpperSaturationLimit=1  LowerSaturationLimit=-1  LinearizeAsGain=on  AntiWindupMode=clamping  Kb=1  POutMin=[]  POutMax=[]  IOutMin=[]  IOutMax=[]  DOutMin=[]  DOutMax=[]  NOutMin=[]  NOutMax=[]  SumOutMin=[]  SumOutMax=[]  SaturationOutMin=[]  SaturationOutMax=[]  PParamMin=[]  PParamMax=[]  IParamMin=[]  IParamMax=[]  DParamMin=[]  DParamMax=[]  NParamMin=[]  NParamMax=[]  KbParamMin=[]  KbParamMax=[]  KtParamMin=[]  KtParamMax=[]  KbOutMin=[]  KbOutMax=[]  KtOutMin=[]  KtOutMax=[]  IntegratorOutMin=[]  IntegratorOutMax=[]  FilterOutMin=[]  FilterOutMax=[]  SumI1OutMin=[]  SumI1OutMax=[]  SumI2OutMin=[]  SumI2OutMax=[]  SumI3OutMin=[]  SumI3OutMax=[]  SumI4OutMin=[]  SumI4OutMax=[]  SumDOutMin=[]  SumDOutMax=[]  DifferentiatorOutMin=[]  DifferentiatorOutMax=[]  FilterDiffOutCoefMin=[]  FilterDiffOutCoefMax=[]  ReciprocalOutMin=[]  ReciprocalOutMax=[]  SumDenOutMin=[]  SumDenOutMax=[]  SumNumOutMin=[]  SumNumOutMax=[]  DivideOutMin=[]  DivideOutMax=[]  UdiffTsProdOutMin=[]  UdiffTsProdOutMax=[]  NTsProdOutMin=[]  NTsProdOutMax=[]  UintegralTsProdOutMin=[]  UintegralTsProdOutMax=[]  UngainTsProdOutMin=[]  UngainTsProdOutMax=[]  IntegratorContinuousStateAttributes=''  IntegratorStateMustResolveToSignalObject=off  IntegratorRTWStateStorageClass=Auto  FilterContinuousStateAttributes=''  FilterStateMustResolveToSignalObject=off  FilterRTWStateStorageClass=Auto  ParallelPVariant=InternalParameters  IdealPVariant=Disabled  IVariant=InternalParameters  DVariant=InternalParameters  IntegratorVariant=Discrete  SatVariant=Enabled  AWVariant=DiscClampingParallel  PCopyVariant=Disabled  TRVariant=Disabled  FdbkBlocksVariant=Forward  IdealPFdbkVariant=Disabled  SatFdbkVariant=Disabled  DerivativeFilterVariant=ForwardEulerFilter  NVariant=InternalParameters  NCopyVariant=Disabled  FilterICVariant=InternalICsFilter  IntegratorICVariant=InternalICs  ExternalResetVariant=Disabled  TRSumVariant=Passthrough  SumFdbkVariant=Disabled  SumVariant=Sum_PID  TsampFilterVariant=InternalTs  TsampNgainVariant=Passthrough  TsampIntegralVariant=Passthrough  ExternalSaturationOutDataTypeStr=Inherit: Same as second input
  Sqrt : Sqrt  SaturateOnIntegerOverflow=on
  Square : Math  Operator=square  SaturateOnIntegerOverflow=on
  Sum : Sum  Inputs=+
  Sum1 : Sum  Inputs=+-
  Terminator : Terminator
  driver_input : Outport
  wires:
  In1/1 -> driver_input/1, Sum1/1
  Sum1/1 -> PID Controller/1
  Sqrt/1 -> Sum1/2
  Square/1 -> Sum/1
  Sum/1 -> Sqrt/1
  Mux/1 -> Square/1
  VB CoG Y-Velocity/1 -> Mux/2
  VB CoG X-Velocity/1 -> Mux/1
  PID Controller/1 -> Terminator/1

== system Vehicle_Model_Controller_Feb25/Driver Input Logic/ Wheel Velocities ==
  Info Bus : Inport
  Bus Selector1 : BusSelector  OutputSignals=BdyFrm.FrntAxl.Lft.Vel.xdot,BdyFrm.FrntAxl.Lft.Vel.ydot,BdyFrm.FrntAxl.Rght.Vel.xdot,BdyFrm.FrntAxl.Rght.Vel.ydot,BdyFrm.RearAxl.Lft.Vel.xdot,BdyFrm.RearAxl.Rght.Vel.xdot
  Mux : Mux  Inputs=6
  Wheel Velocities : Outport
  wires:
  Mux/1 -> Wheel Velocities/1
  Bus Selector1/4 -> Mux/4  "<ydot>"
  Bus Selector1/2 -> Mux/2  "<ydot>"
  Bus Selector1/6 -> Mux/6  "<xdot>"
  Bus Selector1/5 -> Mux/5  "<xdot>"
  Bus Selector1/3 -> Mux/3  "<xdot>"
  Bus Selector1/1 -> Mux/1  "<xdot>"
  Info Bus/1 -> Bus Selector1/1

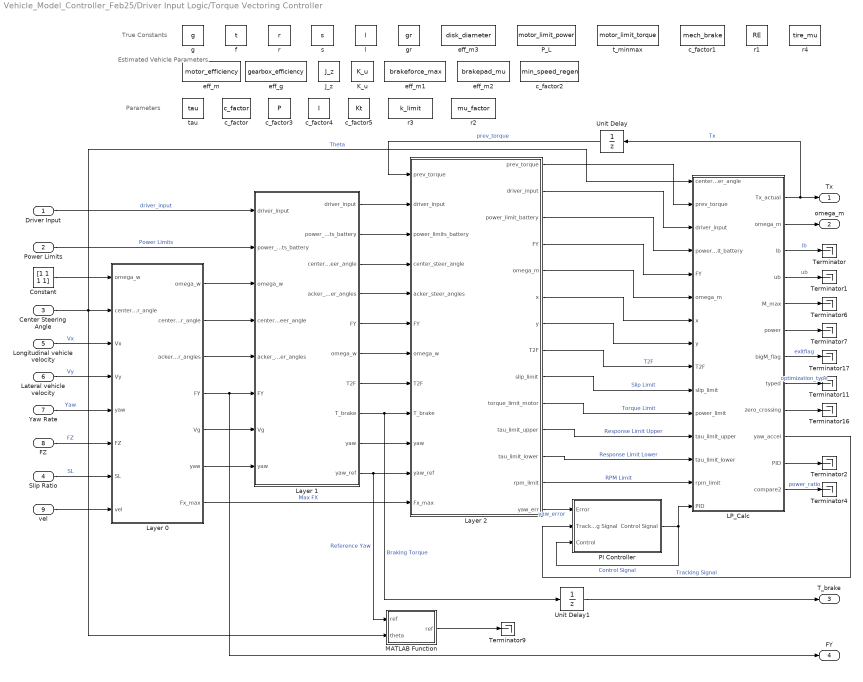
== system Vehicle_Model_Controller_Feb25/Driver Input Logic/Torque Vectoring Controller ==
  note: Parameters
  note: Estimated Vehicle
      | Parameters
  note: True Constants
  Driver Input : Inport
  Power Limits : Inport  Port=2
  Center Steering Angle : Inport  Port=3
  Slip Ratio : Inport  Port=4
  Longitudinal vehicle velocity : Inport  Port=5
  Lateral vehicle velocity : Inport  Port=6
  Yaw Rate : Inport  Port=7
  FZ : Inport  Port=8
  vel : Inport  Port=9
  Constant : Constant  Value=[1 1 1 1]  VectorParams1D=off
  J_z : DataStoreMemory  Description=Polar moment of inertia [kg m^2]  DataStoreName=J_z  ReadBeforeWriteMsg=warning  WriteAfterWriteMsg=warning  WriteAfterReadMsg=warning  InitialValue=150  VectorParams1D=off  ShowAdditionalParam=off  OutDataTypeStr=double
  K_u : DataStoreMemory  Description=Understeer Gradient [rad/m/s^2]  DataStoreName=K_u  ReadBeforeWriteMsg=warning  WriteAfterWriteMsg=warning  WriteAfterReadMsg=warning  InitialValue=0.06  VectorParams1D=off  ShowAdditionalParam=off  OutDataTypeStr=double
  "LP_Calc " : MATLAB Function  TreatAsAtomicUnit=on
  Layer 0 : MATLAB Function  TreatAsAtomicUnit=on
  Layer 1 : MATLAB Function  TreatAsAtomicUnit=on
  Layer 2 : MATLAB Function  TreatAsAtomicUnit=on
  MATLAB Function : MATLAB Function  TreatAsAtomicUnit=on
  PI Controller : Subsystem
  P_L : DataStoreMemory  Description=Power limit for each motor [W]  DataStoreName=motor_limit_power  ReadBeforeWriteMsg=warning  WriteAfterWriteMsg=warning  WriteAfterReadMsg=warning  InitialValue=[15000, 15000, 15000, 15000]  VectorParams1D=off  ShowAdditionalParam=off  OutDataTypeStr=double  Dimensions=[1 4]
  Terminator{,1..2,4,6..7,9,11,16..17} (10 alike) : Terminator
  Unit Delay : UnitDelay  InitialCondition=[0; 0; 0; 0]  SampleTime=-1  HasFrameUpgradeWarning=on
  Unit Delay1 : UnitDelay  InitialCondition=[0, 0, 0, 0]  SampleTime=-1  HasFrameUpgradeWarning=on
  c_factor : DataStoreMemory  Description=Max yaw equation contributing factor [Unitless]  DataStoreName=c_factor  ReadBeforeWriteMsg=warning  WriteAfterWriteMsg=warning  WriteAfterReadMsg=warning  InitialValue=0.8  VectorParams1D=off  ShowAdditionalParam=off  OutDataTypeStr=double
  c_factor1 : DataStoreMemory  Description=The value of driver_input where mechanical braking begins [Unitless]  DataStoreName=mech_brake  ReadBeforeWriteMsg=warning  WriteAfterWriteMsg=warning  WriteAfterReadMsg=warning  InitialValue=-0.5  VectorParams1D=off  ShowAdditionalParam=off  OutDataTypeStr=double
  c_factor2 : DataStoreMemory  Description=Minimum motor shaft rotation rate for regenerative braking [Unitless]  DataStoreName=min_speed_regen  ReadBeforeWriteMsg=warning  WriteAfterWriteMsg=warning  WriteAfterReadMsg=warning  InitialValue=85  VectorParams1D=off  ShowAdditionalParam=off  OutDataTypeStr=double
  c_factor3 : DataStoreMemory  Description=Proportional gain of PI controller  DataStoreName=P  ReadBeforeWriteMsg=warning  WriteAfterWriteMsg=warning  WriteAfterReadMsg=warning  InitialValue=3.07  VectorParams1D=off  ShowAdditionalParam=off  OutDataTypeStr=double
  c_factor4 : DataStoreMemory  Description=Integral gain of PI controller  DataStoreName=I  ReadBeforeWriteMsg=warning  WriteAfterWriteMsg=warning  WriteAfterReadMsg=warning  InitialValue=6.74  VectorParams1D=off  ShowAdditionalParam=off  OutDataTypeStr=double
  c_factor5 : DataStoreMemory  Description=Integral gain of PI controller  DataStoreName=Kt  ReadBeforeWriteMsg=warning  WriteAfterWriteMsg=warning  WriteAfterReadMsg=warning  InitialValue=5.56  VectorParams1D=off  ShowAdditionalParam=off  OutDataTypeStr=double
  eff_g : DataStoreMemory  Description=Gearbox power transmission efficiency [Unitless]  DataStoreName=gearbox_efficiency  ReadBeforeWriteMsg=warning  WriteAfterWriteMsg=warning  WriteAfterReadMsg=warning  InitialValue=[0.97 0.97 0.97 0.97]  VectorParams1D=off  ShowAdditionalParam=off  OutDataTypeStr=double
  eff_m : DataStoreMemory  Description=Motor efficiency [Unitless]  DataStoreName=motor_efficiency  ReadBeforeWriteMsg=warning  WriteAfterWriteMsg=warning  WriteAfterReadMsg=warning  InitialValue=[0.85, 0.85, 0.85, 0.85]  VectorParams1D=off  ShowAdditionalParam=off  OutDataTypeStr=double  Dimensions=[1 4]
  eff_m1 : DataStoreMemory  Description=Max force brakes can exert on each wheel [N]  DataStoreName=brakeforce_max  ReadBeforeWriteMsg=warning  WriteAfterWriteMsg=warning  WriteAfterReadMsg=warning  InitialValue=[250,250,250,250]  VectorParams1D=off  ShowAdditionalParam=off  OutDataTypeStr=double  Dimensions=[1 4]
  eff_m2 : DataStoreMemory  Description=brakepad friction coefficient[Unitless]  DataStoreName=brakepad_mu  ReadBeforeWriteMsg=warning  WriteAfterWriteMsg=warning  WriteAfterReadMsg=warning  InitialValue=[0.5,0.5,0.5,0.5]  VectorParams1D=off  ShowAdditionalParam=off  OutDataTypeStr=double  Dimensions=[1 4]
  eff_m3 : DataStoreMemory  Description=Diameter of brake disk [m]  DataStoreName=disk_diameter  ReadBeforeWriteMsg=warning  WriteAfterWriteMsg=warning  WriteAfterReadMsg=warning  InitialValue=[0.1,0.1,0.1,0.1]  VectorParams1D=off  ShowAdditionalParam=off  OutDataTypeStr=double  Dimensions=[1 4]
  f : DataStoreMemory  Description=controller timing [s]  DataStoreName=t  ReadBeforeWriteMsg=warning  WriteAfterWriteMsg=warning  WriteAfterReadMsg=warning  InitialValue=0.015  VectorParams1D=off  ShowAdditionalParam=off  OutDataTypeStr=double
  g : DataStoreMemory  Description=acceleration due to gravity [m/s^2]  DataStoreName=g  ReadBeforeWriteMsg=warning  WriteAfterWriteMsg=warning  WriteAfterReadMsg=warning  InitialValue=9.81  VectorParams1D=off  ShowAdditionalParam=off  OutDataTypeStr=double
  gr : DataStoreMemory  Description=Gear ratios [Unitless]  DataStoreName=gr  ReadBeforeWriteMsg=warning  WriteAfterWriteMsg=warning  WriteAfterReadMsg=warning  InitialValue=[6.63043, 6.63043, 7.95652, 7.95652]  VectorParams1D=off  ShowAdditionalParam=off  OutDataTypeStr=double  Dimensions=[1 4]
  l : DataStoreMemory  Description=Wheelbase [m]  DataStoreName=l  ReadBeforeWriteMsg=warning  WriteAfterWriteMsg=warning  WriteAfterReadMsg=warning  InitialValue=[0.7922471, 0.7828529]  VectorParams1D=off  ShowAdditionalParam=off  OutDataTypeStr=double  Dimensions=[1 2]
  r : DataStoreMemory  Description=Tire radius [m]  DataStoreName=r  ReadBeforeWriteMsg=warning  WriteAfterWriteMsg=warning  WriteAfterReadMsg=warning  InitialValue=0.22  VectorParams1D=off  ShowAdditionalParam=off  OutDataTypeStr=double
  r1 : DataStoreMemory  Description=Tire radius [m]  DataStoreName=RE  ReadBeforeWriteMsg=warning  WriteAfterWriteMsg=warning  WriteAfterReadMsg=warning  InitialValue=0.2228169203  VectorParams1D=off  ShowAdditionalParam=off  OutDataTypeStr=double
  r2 : DataStoreMemory  Description=Tire radius [m]  DataStoreName=mu_factor  ReadBeforeWriteMsg=warning  WriteAfterWriteMsg=warning  WriteAfterReadMsg=warning  InitialValue=2/3  VectorParams1D=off  ShowAdditionalParam=off  OutDataTypeStr=double
  r3 : DataStoreMemory  Description=Tire radius [m]  DataStoreName=k_limit  ReadBeforeWriteMsg=warning  WriteAfterWriteMsg=warning  WriteAfterReadMsg=warning  InitialValue=3  VectorParams1D=off  ShowAdditionalParam=off  OutDataTypeStr=double
  r4 : DataStoreMemory  Description=Tire radius [m]  DataStoreName=tire_mu  ReadBeforeWriteMsg=warning  WriteAfterWriteMsg=warning  WriteAfterReadMsg=warning  InitialValue=0.8  VectorParams1D=off  ShowAdditionalParam=off  OutDataTypeStr=double
  s : DataStoreMemory  Description=Half track width [m]  DataStoreName=s  ReadBeforeWriteMsg=warning  WriteAfterWriteMsg=warning  WriteAfterReadMsg=warning  InitialValue=[0.647895, 0.62102]  VectorParams1D=off  ShowAdditionalParam=off  OutDataTypeStr=double  Dimensions=[1 2]
  t_minmax : DataStoreMemory  Description=Minimum and maximum torque request from motor [Nm]  DataStoreName=motor_limit_torque  ReadBeforeWriteMsg=warning  WriteAfterWriteMsg=warning  WriteAfterReadMsg=warning  InitialValue=[-25, 25]  VectorParams1D=off  ShowAdditionalParam=off  OutDataTypeStr=double  Dimensions=[1 2]
  tau : DataStoreMemory  Description=Motor Response Time Constant [s]  DataStoreName=tau  ReadBeforeWriteMsg=warning  WriteAfterWriteMsg=warning  WriteAfterReadMsg=warning  InitialValue=0.1  VectorParams1D=off  ShowAdditionalParam=off  OutDataTypeStr=double
  Tx : Outport
  omega_m : Outport  Port=2
  T_brake : Outport  Port=3
  FY : Outport  Port=4
  wires:
  Driver Input/1 -> Layer 1/1("driver_input ")  "driver_input"
  Layer 1/7(T2F) -> Layer 2/8("T2F ")
  Layer 2/14(yaw_err) -> PI Controller/1(Error)  "yaw_error"
  Layer 2/10(torque_limit_motor) -> "LP_Calc "/11(power_limit)  "Torque Limit"
  Power Limits/1 -> Layer 1/2("power_limits_battery ")  "Power Limits"
  Layer 0/6(yaw) -> Layer 1/8("yaw ")
  Layer 1/3(center_steer_angle) -> Layer 2/4(center_steer_angle)
  Layer 1/4(acker_steer_angles) -> Layer 2/5(acker_steer_angles)
  Layer 1/6(omega_w) -> Layer 2/7(omega_w)
  Layer 2/6(x) -> "LP_Calc "/7(x)
  Layer 2/9(slip_limit) -> "LP_Calc "/10(slip_limit)  "Slip Limit"
  Layer 1/5(FY) -> Layer 2/6("FY ")
  Layer 0/5(Vg) -> Layer 1/7(Vg)
  Layer 0/3(acker_steer_angles) -> Layer 1/5("acker_steer_angles ")
  Layer 2/3(power_limit_battery) -> "LP_Calc "/4(power_limit_battery)
  Layer 0/2(center_steer_angle) -> Layer 1/4("center_steer_angle ")
  Layer 1/10(yaw_ref) -> MATLAB Function/1("ref "), Layer 2/11(yaw_ref)  "Reference Yaw"
  Layer 2/7(y) -> "LP_Calc "/8(y)
  Layer 2/2(driver_input) -> "LP_Calc "/3(driver_input)
  Layer 2/4(FY) -> "LP_Calc "/5(FY)
  Layer 1/9(yaw) -> Layer 2/10(yaw)
  Layer 1/1(driver_input) -> Layer 2/2("driver_input ")
  Layer 1/2(power_limits_battery) -> Layer 2/3(power_limits_battery)
  Layer 2/8(T2F) -> "LP_Calc "/9(T2F)  "T2F"
  Unit Delay/1 -> Layer 2/1("prev_torque ")  "prev_torque"
  Layer 2/11(tau_limit_upper) -> "LP_Calc "/12(tau_limit_upper)  "Response Limit Upper"
  Layer 2/12(tau_limit_lower) -> "LP_Calc "/13(tau_limit_lower)  "Response Limit Lower"
  "LP_Calc "/3(lb) -> Terminator/1  "lb"
  "LP_Calc "/4(ub) -> Terminator1/1  "ub"
  Layer 2/1(prev_torque) -> "LP_Calc "/2(prev_torque)
  "LP_Calc "/2(omega_m) -> omega_m/1
  "LP_Calc "/5(M_max) -> Terminator6/1
  Layer 1/8(T_brake) -> Layer 2/9(T_brake), Unit Delay1/1  "Braking Torque"
  PI Controller/1(Control Signal) -> PI Controller/3(Control), "LP_Calc "/15("PID ")  "Control Signal"
  Unit Delay1/1 -> T_brake/1
  "LP_Calc "/10(yaw_accel) -> PI Controller/2(Tracking Signal)  "Tracking Signal"
  FZ/1 -> Layer 0/6(FZ)  "FZ"
  Longitudinal vehicle velocity/1 -> Layer 0/3(Vx)  "Vx"
  Yaw Rate/1 -> Layer 0/5("yaw ")  "Yaw"
  Constant/1 -> Layer 0/1("omega_w ")
  Lateral vehicle velocity/1 -> Layer 0/4(Vy)  "Vy"
  Center Steering Angle/1 -> MATLAB Function/2(theta), Layer 0/2("center_steer_angle "), "LP_Calc "/1(center_steer_angle)  "Theta"
  Layer 0/1(omega_w) -> Layer 1/3("omega_w ")
  vel/1 -> Layer 0/8(vel)
  Layer 0/4(FY) -> FY/1, Layer 1/6("FY ")
  Layer 0/7(Fx_max) -> Layer 2/12(Fx_max)  "Max FX"
  Layer 2/13(rpm_limit) -> "LP_Calc "/14(rpm_limit)  "RPM Limit"
  "LP_Calc "/6(power) -> Terminator7/1
  "LP_Calc "/7(bigM_flag) -> Terminator17/1  "exitflag"
  "LP_Calc "/8(typed) -> Terminator11/1  "optimization_type"
  "LP_Calc "/9(zero_crossing) -> Terminator16/1
  "LP_Calc "/11(PID) -> Terminator2/1
  Layer 2/5(omega_m) -> "LP_Calc "/6("omega_m ")
  "LP_Calc "/12(compare2) -> Terminator4/1  "power_ratio"
  Slip Ratio/1 -> Layer 0/7(SL)  "SL"
  "LP_Calc "/1(Tx_actual) -> Unit Delay/1, Tx/1  "Tx"
  MATLAB Function/1(ref) -> Terminator9/1

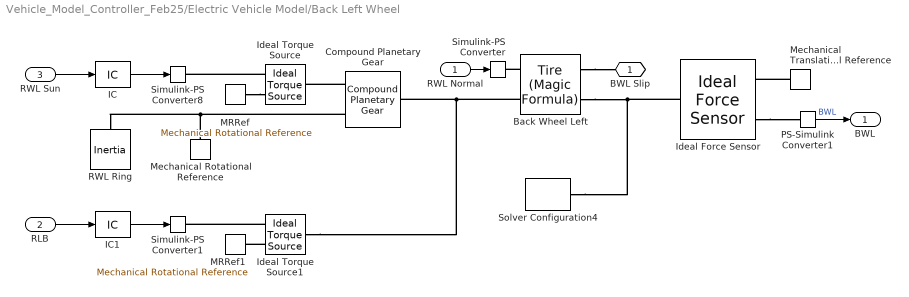
== system Vehicle_Model_Controller_Feb25/Electric Vehicle Model/Back Left Wheel ==
  RWL Normal : Inport
  RLB : Inport  Port=2
  RWL Sun : Inport  Port=3
  Back Wheel Left : sdl_lib/Tires & Vehicles/Tire (Magic Formula)  parameterization=sdl.enum.magic_tire_model.peak  F_z1=1400 N  F_x1=3000 N  kappa1=15  B_m=0.848  C_m=0.19  D_m=5.97  E_m=1.1  fz0=4000 N  p_Cx=1.685  p_Dx=[1.21, -.037]  p_Ex=[.344, .095, -.02, 0]  p_Kx=[21.51, -.163, .245]  p_Hx=[-.002, .002]  p_Vx=[0, 0]  v_tr_thr=0.1 m/s  r_e=0.2228169203 m  model_compliance=0  stiffness=2e5 N/m  damping=1000 N/(m/s)  model_inertia=1  inertia=0.03 kg*m^2  initial_velocity=0 rad/s  model_resistance=0  resistance_model=1  coeff=0.015  p_tire=82.74e3 Pa  alpha=-0.003  beta=0.97  coeff_a=84e-4  coeff_b=6.2e-4 s/m  coeff_c=1.6e-4 s^2/m^2  v_thr=0.01 m/s
  Compound Planetary Gear : sdl_lib/Gears/Compound Planetary Gear  rp_ratio=84/23  ps_ratio=40/21  friction_model=sdl.enum.gear_friction.constant  mu_visc=[0, 0] N*m/(rad/s)  efficiency=[.97, 1]  temperature_TLU=[280, 300, 320] K  efficiency_sp_TLU=[.95, .9, .85]  efficiency_rp_TLU=[.95, .9, .85]  pwr_thr=[.001, .001] W  thermal_mass=50 J/K  T_init=300 K  model_inertia=simscape.enum.onoff.off  planet_inertia=0.001 kg*m^2
      settings: SourceProductBaseCode=LD  InternalSimscapePortConfiguration="{\"Bottom\":[],\"Left\":[{\"id\":\"C\",\"label\":\"C\",\"type\":\"foundation.mechanical.rotational.rotational\"}],\"Right\":[{\"id\":\"R\",\"label\":\"R\",\"type\":\"foundation.mechanical.rotational.rotational\"},{\"id\":\"S\",\"label\":\"S\",\"type\":\"foundation.mechanical.rotational.rotational\"}],\"Top\":[]}"
  IC : InitialCondition  Value=0
  IC1 : InitialCondition  Value=0
  Ideal Force Sensor : fl_lib/Mechanical/Mechanical Sensors/Ideal Force Sensor
  Ideal Torque Source : fl_lib/Mechanical/Mechanical Sources/Ideal Torque Source
      settings: SourceProductName=Foundation Library
  Ideal Torque Source1 : fl_lib/Mechanical/Mechanical Sources/Ideal Torque Source
      settings: SourceProductName=Foundation Library
  MRRef : fl_lib/Mechanical/Rotational Elements/Mechanical Rotational Reference
      settings: SourceProductName=Foundation Library
  MRRef1 : fl_lib/Mechanical/Rotational Elements/Mechanical Rotational Reference
      settings: SourceProductName=Foundation Library
  Mechanical Rotational Reference : fl_lib/Mechanical/Rotational Elements/Mechanical Rotational Reference
  Mechanical Translational Reference : fl_lib/Mechanical/Translational Elements/Mechanical Translational Reference
  PS-Simulink Converter1 : nesl_utility/PS-Simulink Converter  PhysicalDomain=network_engine_domain  SubClassName=ps_output  LeftPortType=input  RightPortType=output  PseudoPeriodic=off  Frequencies=[]  Unit=N  AffineConversion=off
      settings: SourceProductBaseCode=PW,SS
  RWL Ring : fl_lib/Mechanical/Rotational Elements/Inertia  inertia=0.1 kg*m^2  num_ports=foundation.enum.numPorts2.one  w_specify=off  w_priority=High  w=0 rad/s  w_nominal_specify=off  w_nominal_unit=rad/s  w_nominal_value=1  t_specify=off  t_priority=None  t=0 N*m  t_nominal_specify=off  t_nominal_unit=N*m  t_nominal_value=1
  Simulink-PS Converter : nesl_utility/Simulink-PS Converter  PhysicalDomain=network_engine_domain  SubClassName=ps_input  LeftPortType=input  RightPortType=output  PseudoPeriodic=off  Frequencies=[]  NoiseDistribution=none  NoiseParameters=[]  Unit=N  AffineConversion=off  FilteringAndDerivatives=zero  SimscapeFilterOrder=1  InputFilterTimeConstant=0.001  UdotUserProvided=0
      settings: SourceProductBaseCode=PW,SS
  Simulink-PS Converter1 : nesl_utility/Simulink-PS Converter  PhysicalDomain=network_engine_domain  SubClassName=ps_input  LeftPortType=input  RightPortType=output  PseudoPeriodic=off  Frequencies=[]  NoiseDistribution=none  NoiseParameters=[]  Unit=N*m  AffineConversion=off  FilteringAndDerivatives=zero  SimscapeFilterOrder=1  InputFilterTimeConstant=0.001  UdotUserProvided=0
      settings: SourceProductBaseCode=PW,SS
  Simulink-PS Converter8 : nesl_utility/Simulink-PS Converter  PhysicalDomain=network_engine_domain  SubClassName=ps_input  LeftPortType=input  RightPortType=output  PseudoPeriodic=off  Frequencies=[]  NoiseDistribution=none  NoiseParameters=[]  Unit=N*m  AffineConversion=off  FilteringAndDerivatives=zero  SimscapeFilterOrder=1  InputFilterTimeConstant=0.001  UdotUserProvided=0
      settings: SourceProductBaseCode=PW,SS
  Solver Configuration4 : nesl_utility/Solver Configuration  PhysicalDomain=network_engine_domain  SubClassName=solver  LeftPortType=input  RightPortType=generic  Tones=[]  Harmonics=[]  SimulateNoise=off  Profile=off  UseLocalSampling=off  EnableSwitchedLinearOptims=on  FrequencyDomain=off  UseCCode=off  RelTol=0.001  AbsTol=1e-06  MinStep=1e-09  ToWorkspace=off  RevertToSquareIcSolve=off  NumHomotopyIterations=100  PhasorMode=off  PhasorModeNumHarmonics=1  DoDC=off  ResidualTolerance=1e-09  UseLocalSolver=off  LocalSolverChoice=NE_BACKWARD_EULER_ADVANCER  LocalSolverSampleTime=0.001  DoFixedCost=off  MaxNonlinIter=300  MaxModeIter=20  ComputeImpulses=off  ImpulseIterations=2  LinearAlgebra=auto  EquationFormulation=NE_TIME_EF  DelaysMemoryBudget=1024  AutomaticFiltering=off  FilteringTimeConstant=0.001  PartitionStorageMethod=AS_NEEDED  PartitionMemoryBudget=1024  PartitionMethod=ROBUST
      settings: SourceProductBaseCode=PW,SS
  BWL Slip : PMIOPort  Side=Left
  BWL : Outport
  wires:
  PS-Simulink Converter1/1 -> BWL/1  "BWL"
  RWL Normal/1 -> Simulink-PS Converter/1
  IC/1 -> Simulink-PS Converter8/1
  RWL Sun/1 -> IC/1
  IC1/1 -> Simulink-PS Converter1/1
  RLB/1 -> IC1/1
  connections:
  Back Wheel Left/RConn1 -- BWL Slip/RConn1
  Ideal Torque Source1/LConn1 -- Back Wheel Left/LConn2 -- Compound Planetary Gear/LConn1
  Ideal Force Sensor/RConn2 -- PS-Simulink Converter1/LConn1
  Ideal Force Sensor/LConn1 -- Back Wheel Left/RConn2 -- Solver Configuration4/RConn1
  Back Wheel Left/LConn1 -- Simulink-PS Converter/RConn1
  Mechanical Translational Reference/LConn1 -- Ideal Force Sensor/RConn1
  Mechanical Rotational Reference/LConn1 -- RWL Ring/LConn1 -- Compound Planetary Gear/RConn1
  Ideal Torque Source/RConn1 -- Simulink-PS Converter8/RConn1
  Compound Planetary Gear/RConn2 -- Ideal Torque Source/LConn1
  MRRef/LConn1 -- Ideal Torque Source/RConn2
  Ideal Torque Source1/RConn1 -- Simulink-PS Converter1/RConn1
  Ideal Torque Source1/RConn2 -- MRRef1/LConn1
